simulink model "test_decoupling_bus_and_VF_replay"  (R2025b)
settings: Solver=VariableStepAuto  StartTime=0.0  StopTime=20  RelTol=1e-3
undefined symbols (not defined in the file): Circuit, DiscIntNeverNeededParam, Open, Short
libraries: nesl_utility x15, ee_lib_for_power_systems x10, ee_lib x8, simulink x3
settings Model: Creator=gdudgeon  LastModifiedBy=gdudgeon
settings RTWCC: GPUComputeCapability=3.5

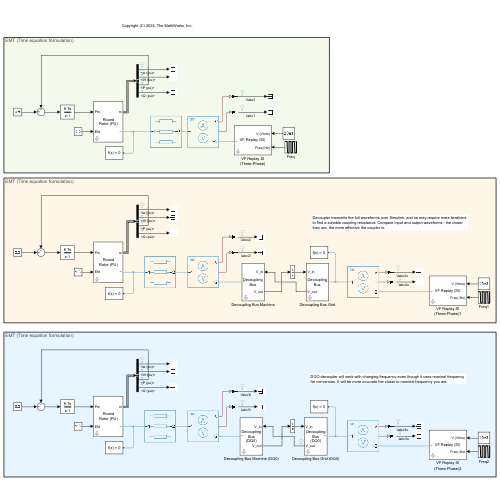
[thumbnail: Simulink's stored preview of the top-level diagram]
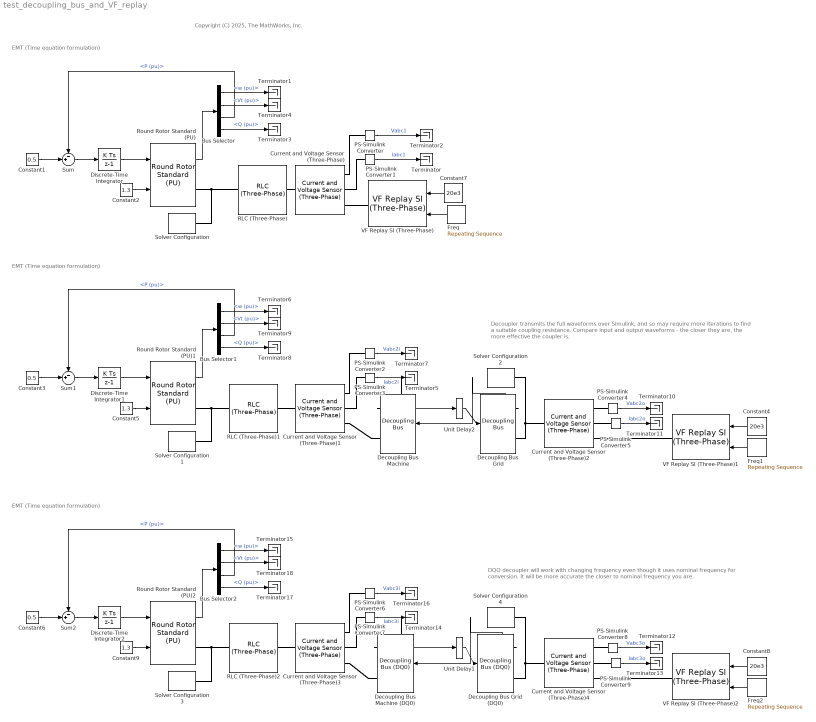
== system test_decoupling_bus_and_VF_replay ==
  note: DQO decoupler will work with changing frequency even though it uses nominal frequency for conversion. It will be more accurate the closer to nominal frequency you are.
  note: EMT (Time equation formulation)
  note: Copyright (C) 2025, The MathWorks, Inc.
  note: EMT (Time equation formulation)
  note: EMT (Time equation formulation)
  note: Decoupler transmits the full waveforms over Simulink, and so may require more iterations to find a suitable coupling resistance. Compare input and output waveforms - the closer they are, the more effective the coupler is.
  Bus Selector : BusSelector  OutputSignals=w (pu),Vt (pu),P (pu),Q (pu)
  Bus Selector1 : BusSelector  OutputSignals=w (pu),Vt (pu),P (pu),Q (pu)
  Bus Selector2 : BusSelector  OutputSignals=w (pu),Vt (pu),P (pu),Q (pu)
  Constant1 : Constant  Value=0.5
  Constant2 : Constant  Value=1.3
  Constant3 : Constant  Value=0.5
  Constant4 : Constant  Value=20e3  SampleTime=-1
  Constant5 : Constant  Value=1.3
  Constant6 : Constant  Value=0.5
  Constant7 : Constant  Value=20e3  SampleTime=-1
  Constant8 : Constant  Value=20e3  SampleTime=-1
  Constant9 : Constant  Value=1.3
  Current and Voltage Sensor (Three-Phase){,1..4} (5 alike) : ee_lib/Sensors & Transducers/Current and Voltage Sensor (Three-Phase)  vMeasurementType=ee.enum.vmeasurement.lg  outputUnit=ee.enum.unit.si  SRated=100e6 A*V  VRated=24e3 V  I_specify=off  I_priority=None  I=[0, 0, 0] A  I_nominal_specify=off  I_nominal_value=1  I_nominal_unit=A  V_specify=off  V_priority=None  V=[0, 0, 0] V  V_nominal_specify=off  V_nominal_value=1  V_nominal_unit=V
      settings: InternalSimscapePortConfiguration="{\"Bottom\":[],\"Left\":[{\"id\":\"N1\",\"label\":\"~1\",\"type\":\"foundation.electrical.three_phase\"}],\"Right\":[{\"id\":\"V_output\",\"label\":\"V\",\"type\":\"output\"},{\"id\":\"I_output\",\"label\":\"I\",\"type\":\"output\"},{\"id\":\"N2\",\"label\":\"~2\",\"type\":\"foundation.electrical.three_phase\"}],\"Top\":[]}"
  Decoupling Bus Grid : ee_lib_for_power_systems/Utilities/Decoupling Bus  Rcouple=100
      settings: SourceProductName=Support Library for Power Systems
  Decoupling Bus Grid (DQ0) : ee_lib_for_power_systems/Utilities/Decoupling Bus (DQ0)  Rcouple=10  freq=60
      settings: SourceProductName=Support Library for Power Systems
  Decoupling Bus Machine : ee_lib_for_power_systems/Utilities/Decoupling Bus  Rcouple=100
      settings: SourceProductName=Support Library for Power Systems
  Decoupling Bus Machine (DQ0) : ee_lib_for_power_systems/Utilities/Decoupling Bus (DQ0)  Rcouple=10  freq=60
      settings: SourceProductName=Support Library for Power Systems
  Discrete-Time Integrator : DiscreteIntegrator  gainval=1  SampleTime=-1  ICPrevOutput=DiscIntNeverNeededParam  ICPrevScaledInput=DiscIntNeverNeededParam
  Discrete-Time Integrator1 : DiscreteIntegrator  gainval=1  SampleTime=-1  ICPrevOutput=DiscIntNeverNeededParam  ICPrevScaledInput=DiscIntNeverNeededParam
  Discrete-Time Integrator2 : DiscreteIntegrator  gainval=1  SampleTime=-1  ICPrevOutput=DiscIntNeverNeededParam  ICPrevScaledInput=DiscIntNeverNeededParam
  Freq : simulink/Sources/Repeating Sequence  rep_seq_t=[0 10 12 20]  rep_seq_y=[1 1 0.95 0.95]*60
  Freq1 : simulink/Sources/Repeating Sequence  rep_seq_t=[0 10 12 20]  rep_seq_y=[1 1 0.95 0.95]*60
  Freq2 : simulink/Sources/Repeating Sequence  rep_seq_t=[0 10 12 20]  rep_seq_y=[1 1 0.95 0.95]*60
  PS-Simulink Converter{,1..9} (10 alike) : nesl_utility/PS-Simulink Converter  PhysicalDomain=network_engine_domain  SubClassName=ps_output  LeftPortType=input  RightPortType=output  PseudoPeriodic=off  Frequencies=[]  VectorFormat=inherit  Unit=inherit  AffineConversion=off
  RLC (Three-Phase) : ee_lib/Passive/RLC Assemblies/RLC (Three-Phase)  port_option=ee.enum.threePhasePort.composite  component_structure=ee.enum.rlc.structure.SeriesRL  R=1e-4 Ohm  L=1e-4 H  C=1e-6 F  R_parasitic=0 Ohm  G_parasitic=0 1/Ohm  IL_specify=off  IL_priority=High  IL=[0, 0, 0] A  IL_nominal_specify=off  IL_nominal_value=1  IL_nominal_unit=A  VC_specify=off  VC_priority=High  VC=[0, 0, 0] V  VC_nominal_specify=off  VC_nominal_value=1  VC_nominal_unit=V
      settings: InternalSimscapePortConfiguration="{\"Bottom\":[],\"Left\":[{\"id\":\"N1\",\"label\":\"~1\",\"type\":\"foundation.electrical.three_phase\"}],\"Right\":[{\"id\":\"N2\",\"label\":\"~2\",\"type\":\"foundation.electrical.three_phase\"}],\"Top\":[]}"
  RLC (Three-Phase)1 : ee_lib/Passive/RLC Assemblies/RLC (Three-Phase)  port_option=ee.enum.threePhasePort.composite  component_structure=ee.enum.rlc.structure.SeriesRL  R=1e-4 Ohm  L=1e-4 H  C=1e-6 F  R_parasitic=0 Ohm  G_parasitic=0 1/Ohm  IL_specify=off  IL_priority=High  IL=[0, 0, 0] A  IL_nominal_specify=off  IL_nominal_value=1  IL_nominal_unit=A  VC_specify=off  VC_priority=High  VC=[0, 0, 0] V  VC_nominal_specify=off  VC_nominal_value=1  VC_nominal_unit=V
      settings: InternalSimscapePortConfiguration="{\"Bottom\":[],\"Left\":[{\"id\":\"N1\",\"label\":\"~1\",\"type\":\"foundation.electrical.three_phase\"}],\"Right\":[{\"id\":\"N2\",\"label\":\"~2\",\"type\":\"foundation.electrical.three_phase\"}],\"Top\":[]}"
  RLC (Three-Phase)2 : ee_lib/Passive/RLC Assemblies/RLC (Three-Phase)  port_option=ee.enum.threePhasePort.composite  component_structure=ee.enum.rlc.structure.SeriesRL  R=1e-4 Ohm  L=1e-4 H  C=1e-6 F  R_parasitic=0 Ohm  G_parasitic=0 1/Ohm  IL_specify=off  IL_priority=High  IL=[0, 0, 0] A  IL_nominal_specify=off  IL_nominal_value=1  IL_nominal_unit=A  VC_specify=off  VC_priority=High  VC=[0, 0, 0] V  VC_nominal_specify=off  VC_nominal_value=1  VC_nominal_unit=V
      settings: InternalSimscapePortConfiguration="{\"Bottom\":[],\"Left\":[{\"id\":\"N1\",\"label\":\"~1\",\"type\":\"foundation.electrical.three_phase\"}],\"Right\":[{\"id\":\"N2\",\"label\":\"~2\",\"type\":\"foundation.electrical.three_phase\"}],\"Top\":[]}"
  Round Rotor Standard (PU) : ee_lib_for_power_systems/Electromechanical Machines/Round Rotor Standard (PU)  Pnom=1e6  Vnom=20e3  Fnom=60  Xd=1.5  Xdp=0.4  Xdpp=0.25  Xq=1.4  Xqp=0.5  Xqpp=0.25  Xl=0.1  Ra=0.05  D_Q=[Short-Circuit Open-Circuit]  Tdp=1.2  Tdpp=0.05  Tdop=7  Tdopp=0.05  Tqp=1  Tqpp=0.05  Tqop=1  Tqopp=0.04  H=0.2  D=0  p=4
      settings: SourceProductName=Support Library for Power Systems
  Round Rotor Standard (PU)1 : ee_lib_for_power_systems/Electromechanical Machines/Round Rotor Standard (PU)  Pnom=1e6  Vnom=20e3  Fnom=60  Xd=1.5  Xdp=0.4  Xdpp=0.25  Xq=1.4  Xqp=0.5  Xqpp=0.25  Xl=0.1  Ra=0.05  D_Q=[Short-Circuit Open-Circuit]  Tdp=1.2  Tdpp=0.05  Tdop=7  Tdopp=0.05  Tqp=1  Tqpp=0.05  Tqop=1  Tqopp=0.04  H=0.2  D=0  p=4
      settings: SourceProductName=Support Library for Power Systems
  Round Rotor Standard (PU)2 : ee_lib_for_power_systems/Electromechanical Machines/Round Rotor Standard (PU)  Pnom=1e6  Vnom=20e3  Fnom=60  Xd=1.5  Xdp=0.4  Xdpp=0.25  Xq=1.4  Xqp=0.5  Xqpp=0.25  Xl=0.1  Ra=0.05  D_Q=[Short-Circuit Open-Circuit]  Tdp=1.2  Tdpp=0.05  Tdop=7  Tdopp=0.05  Tqp=1  Tqpp=0.05  Tqop=1  Tqopp=0.04  H=0.2  D=0  p=4
      settings: SourceProductName=Support Library for Power Systems
  "Solver Configuration " : nesl_utility/Solver Configuration  PhysicalDomain=network_engine_domain  SubClassName=solver  LeftPortType=input  RightPortType=generic  Tones=[]  Harmonics=[]  SimulateNoise=off  Profile=off  UseLocalSampling=off  EnableSwitchedLinearOptims=on  FrequencyDomain=off  UseCCode=off  RelTol=0.001  AbsTol=0.001  MinStep=1e-09  ToWorkspace=off  RevertToSquareIcSolve=off  NumHomotopyIterations=100  PhasorMode=off  PhasorModeNumHarmonics=1  ConsistencySolver=NEWTON_XTOL_AFTER_FTOL  IndexReductionMethod=None  DoDC=off  ResidualTolerance=1e-09  ConsistencyTolSource=GLOBAL  ConsistencyAbsTol=0.001  ConsistencyRelTol=0.001  ConsistencyTolFactor=0.001  UseLocalSolver=on  LocalSolverChoice=NE_BACKWARD_EULER_ADVANCER  ResolveIndetEquations=off  FunctionEvalNumThread=1  LocalSolverSampleTime=50e-6  DoFixedCost=off  MaxNonlinIter=2  MaxModeIter=2  ComputeImpulses=off  ImpulseIterations=2  LinearAlgebra=Sparse  LinearAlgebraNumThread=0  EquationFormulation=NE_TIME_EF  DelaysMemoryBudget=1024  AutomaticFiltering=off  FilteringTimeConstant=0.001  PartitionStorageMethod=AS_NEEDED  PartitionMemoryBudget=1024  PartitionMethod=ROBUST  MultibodyUseLocalSolver=off  MultibodyLocalSolverChoice=ODE1  MultibodyLocalSolverSampleTime=0.001
  Solver Configuration {1..4} (4 alike) : nesl_utility/Solver Configuration  PhysicalDomain=network_engine_domain  SubClassName=solver  LeftPortType=input  RightPortType=generic  Tones=[]  Harmonics=[]  SimulateNoise=off  Profile=off  UseLocalSampling=off  EnableSwitchedLinearOptims=on  FrequencyDomain=off  UseCCode=off  RelTol=0.001  AbsTol=0.001  MinStep=1e-09  ToWorkspace=off  RevertToSquareIcSolve=off  NumHomotopyIterations=100  PhasorMode=off  PhasorModeNumHarmonics=1  ConsistencySolver=NEWTON_XTOL_AFTER_FTOL  IndexReductionMethod=None  DoDC=off  ResidualTolerance=1e-09  ConsistencyTolSource=GLOBAL  ConsistencyAbsTol=0.001  ConsistencyRelTol=0.001  ConsistencyTolFactor=0.001  UseLocalSolver=on  LocalSolverChoice=NE_BACKWARD_EULER_ADVANCER  ResolveIndetEquations=off  FunctionEvalNumThread=1  LocalSolverSampleTime=50e-6  DoFixedCost=off  MaxNonlinIter=3  MaxModeIter=2  ComputeImpulses=off  ImpulseIterations=2  LinearAlgebra=Sparse  LinearAlgebraNumThread=0  EquationFormulation=NE_TIME_EF  DelaysMemoryBudget=1024  AutomaticFiltering=off  FilteringTimeConstant=0.001  PartitionStorageMethod=AS_NEEDED  PartitionMemoryBudget=1024  PartitionMethod=ROBUST  MultibodyUseLocalSolver=off  MultibodyLocalSolverChoice=ODE1  MultibodyLocalSolverSampleTime=0.001
  Sum : Sum  Inputs=-+|
  Sum1 : Sum  Inputs=-+|
  Sum2 : Sum  Inputs=-+|
  Terminator{,1..18} (19 alike) : Terminator
  Unit Delay1 : UnitDelay  SampleTime=5e-5  HasFrameUpgradeWarning=on
  Unit Delay2 : UnitDelay  SampleTime=5e-5  HasFrameUpgradeWarning=on
  VF Replay SI (Three-Phase) : ee_lib_for_power_systems/Utilities/VF Replay SI (Three-Phase)  Ts=5e-5
      settings: SourceProductName=Support Library for Power Systems
  VF Replay SI (Three-Phase)1 : ee_lib_for_power_systems/Utilities/VF Replay SI (Three-Phase)  Ts=5e-5
      settings: SourceProductName=Support Library for Power Systems
  VF Replay SI (Three-Phase)2 : ee_lib_for_power_systems/Utilities/VF Replay SI (Three-Phase)  Ts=5e-5
      settings: SourceProductName=Support Library for Power Systems
  wires:
  Round Rotor Standard (PU)/1 -> Bus Selector/1
  Constant1/1 -> Sum/2
  Bus Selector/3 -> Sum/1  "<P (pu)>"
  Bus Selector/4 -> Terminator3/1  "<Q (pu)>"
  Constant7/1 -> VF Replay SI (Three-Phase)/1
  Freq/1 -> VF Replay SI (Three-Phase)/2
  Discrete-Time Integrator/1 -> Round Rotor Standard (PU)/1
  Sum/1 -> Discrete-Time Integrator/1
  Bus Selector/1 -> Terminator1/1  "<w (pu)>"
  PS-Simulink Converter1/1 -> Terminator/1  "Iabc1"
  PS-Simulink Converter/1 -> Terminator2/1  "Vabc1"
  Constant2/1 -> Round Rotor Standard (PU)/2
  Bus Selector/2 -> Terminator4/1  "<Vt (pu)>"
  Bus Selector1/2 -> Terminator9/1  "<Vt (pu)>"
  Constant5/1 -> Round Rotor Standard (PU)1/2
  PS-Simulink Converter2/1 -> Terminator7/1  "Vabc2i"
  PS-Simulink Converter3/1 -> Terminator5/1  "Iabc2i"
  Bus Selector1/1 -> Terminator6/1  "<w (pu)>"
  Sum1/1 -> Discrete-Time Integrator1/1
  Discrete-Time Integrator1/1 -> Round Rotor Standard (PU)1/1
  Freq1/1 -> VF Replay SI (Three-Phase)1/2
  Constant4/1 -> VF Replay SI (Three-Phase)1/1
  Bus Selector1/4 -> Terminator8/1  "<Q (pu)>"
  Bus Selector1/3 -> Sum1/1  "<P (pu)>"
  Constant3/1 -> Sum1/2
  Round Rotor Standard (PU)1/1 -> Bus Selector1/1
  Decoupling Bus Grid/1 -> Decoupling Bus Machine/1
  Decoupling Bus Machine/1 -> Unit Delay2/1
  Unit Delay2/1 -> Decoupling Bus Grid/1
  PS-Simulink Converter4/1 -> Terminator10/1  "Vabc2o"
  PS-Simulink Converter5/1 -> Terminator11/1  "Iabc2o"
  PS-Simulink Converter9/1 -> Terminator13/1  "Iabc3o"
  PS-Simulink Converter8/1 -> Terminator12/1  "Vabc3o"
  Unit Delay1/1 -> Decoupling Bus Grid (DQ0)/1
  Decoupling Bus Machine (DQ0)/1 -> Unit Delay1/1
  Decoupling Bus Grid (DQ0)/1 -> Decoupling Bus Machine (DQ0)/1
  Round Rotor Standard (PU)2/1 -> Bus Selector2/1
  Constant6/1 -> Sum2/2
  Bus Selector2/3 -> Sum2/1  "<P (pu)>"
  Bus Selector2/4 -> Terminator17/1  "<Q (pu)>"
  Constant8/1 -> VF Replay SI (Three-Phase)2/1
  Freq2/1 -> VF Replay SI (Three-Phase)2/2
  Discrete-Time Integrator2/1 -> Round Rotor Standard (PU)2/1
  Sum2/1 -> Discrete-Time Integrator2/1
  Bus Selector2/1 -> Terminator15/1  "<w (pu)>"
  PS-Simulink Converter7/1 -> Terminator14/1  "Iabc3i"
  PS-Simulink Converter6/1 -> Terminator16/1  "Vabc3i"
  Constant9/1 -> Round Rotor Standard (PU)2/2
  Bus Selector2/2 -> Terminator18/1  "<Vt (pu)>"
  connections:
  Round Rotor Standard (PU)/RConn1 -- "Solver Configuration "/RConn1 -- RLC (Three-Phase)/LConn1
  Current and Voltage Sensor (Three-Phase)/LConn1 -- RLC (Three-Phase)/RConn1
  Current and Voltage Sensor (Three-Phase)/RConn3 -- VF Replay SI (Three-Phase)/RConn1
  PS-Simulink Converter/LConn1 -- Current and Voltage Sensor (Three-Phase)/RConn1
  Current and Voltage Sensor (Three-Phase)/RConn2 -- PS-Simulink Converter1/LConn1
  Current and Voltage Sensor (Three-Phase)1/RConn2 -- PS-Simulink Converter3/LConn1
  PS-Simulink Converter2/LConn1 -- Current and Voltage Sensor (Three-Phase)1/RConn1
  Solver Configuration 1/RConn1 -- Round Rotor Standard (PU)1/RConn1 -- RLC (Three-Phase)1/LConn1
  Decoupling Bus Machine/RConn1 -- Current and Voltage Sensor (Three-Phase)1/RConn3
  Solver Configuration 2/RConn1 -- Current and Voltage Sensor (Three-Phase)2/LConn1 -- Decoupling Bus Grid/RConn1
  RLC (Three-Phase)1/RConn1 -- Current and Voltage Sensor (Three-Phase)1/LConn1
  Current and Voltage Sensor (Three-Phase)2/RConn3 -- VF Replay SI (Three-Phase)1/RConn1
  PS-Simulink Converter4/LConn1 -- Current and Voltage Sensor (Three-Phase)2/RConn1
  PS-Simulink Converter5/LConn1 -- Current and Voltage Sensor (Three-Phase)2/RConn2
  Solver Configuration 3/RConn1 -- RLC (Three-Phase)2/LConn1 -- Round Rotor Standard (PU)2/RConn1
  Solver Configuration 4/RConn1 -- Current and Voltage Sensor (Three-Phase)4/LConn1 -- Decoupling Bus Grid (DQ0)/RConn1
  PS-Simulink Converter9/LConn1 -- Current and Voltage Sensor (Three-Phase)4/RConn2
  PS-Simulink Converter8/LConn1 -- Current and Voltage Sensor (Three-Phase)4/RConn1
  Current and Voltage Sensor (Three-Phase)4/RConn3 -- VF Replay SI (Three-Phase)2/RConn1
  Decoupling Bus Machine (DQ0)/RConn1 -- Current and Voltage Sensor (Three-Phase)3/RConn3
  PS-Simulink Converter6/LConn1 -- Current and Voltage Sensor (Three-Phase)3/RConn1
  RLC (Three-Phase)2/RConn1 -- Current and Voltage Sensor (Three-Phase)3/LConn1
  Current and Voltage Sensor (Three-Phase)3/RConn2 -- PS-Simulink Converter7/LConn1
